simulink model "CLSfixedExample3"  (R2025b)
settings: Solver=FixedStepAuto  StartTime=0.0  StopTime=10  FixedStep=0.0005  RelTol=1e-3
undefined symbols (not defined in the file or in its folder): AVI, cfg_length, LRI, pNode_length, pPath_length, PVARP, stepsize, URI, VRP
libraries: Libs x12, Libs_unified x3
settings Model: SimulationMode=accelerator  Creator=ball907  LastModifiedBy=rfen801
settings SolverCC: AutoInsertRateTranBlk=on
settings OptimizationCC: DefaultParameterBehavior=Inlined
settings ModelReferenceCC: EnableRefExpFcnMdlSchedulingChecks=on
settings RTWCC: Toolchain=Simulink Real-Time Toolchain  BuildConfiguration=Faster Runs  CodeExecutionProfiling=on

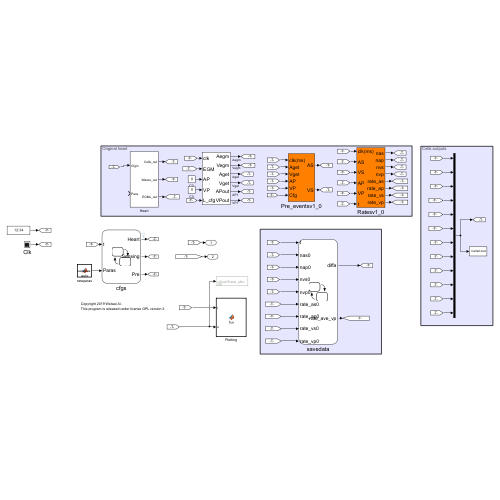
[thumbnail: Simulink's stored preview of the top-level diagram]
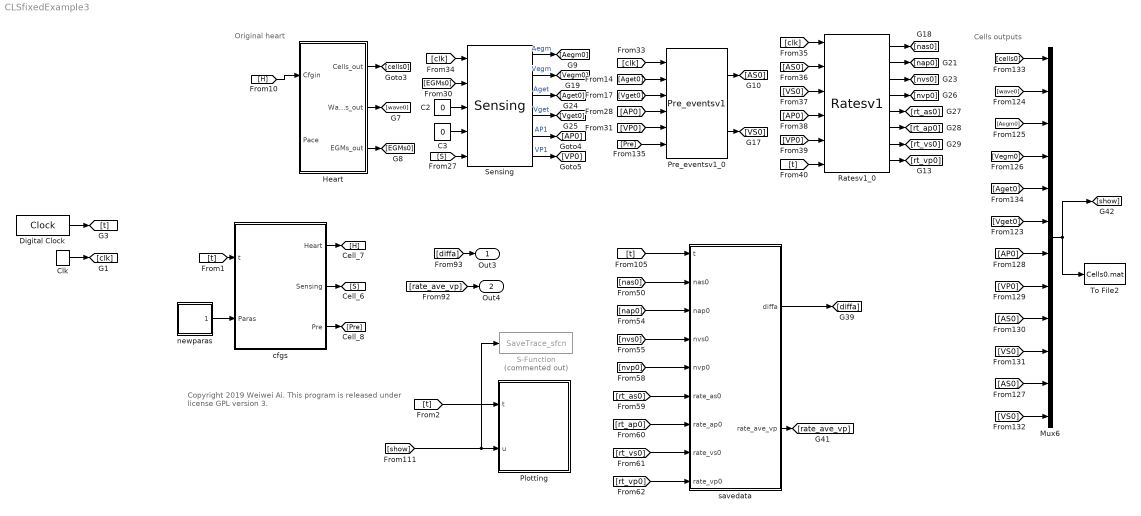
== system CLSfixedExample3 ==
  note: Cells outputs
  note: Copyright 2019 Weiwei Ai.
      | This program is released under license GPL version 3.
  note: Original heart
  C2 : Constant  Value=0
  C3 : Constant  Value=0
  Clk : DiscretePulseGenerator  PulseType=Time based  Period=1  PulseWidth=50
  Digital Clock : DigitalClock  SampleTime=stepsize
  Heart : Subsystem
  Mux6 : Mux  Inputs=12
  Plotting : MATLAB Function  TreatAsAtomicUnit=on  SystemSampleTime=stepsize*5
  Pre_eventsv1_0 : Libs_unified/Pre_eventsv1  SystemSampleTime=-1  VariantActivationTime=update diagram  EmptyChoice=off  PassThrough=off  PassThroughVariantControl=(default)  EmptyChoiceVariantControl=(default)  AllowFlexibleInterface=on  Latency=0  AutoFrameSizeCalculation=off
  Ratesv1_0 : Libs_unified/Ratesv1  SystemSampleTime=-1  VariantActivationTime=update diagram  EmptyChoice=off  PassThrough=off  PassThroughVariantControl=(default)  EmptyChoiceVariantControl=(default)  AllowFlexibleInterface=on  Latency=0  AutoFrameSizeCalculation=off
  S-Function : S-Function  Commented=on  FunctionName=SaveTrace_sfcn  Parameters=1  SFunctionDeploymentMode=off  EnableBusSupport=off
  Sensing : Libs_unified/Sensing  SystemSampleTime=-1  VariantActivationTime=update diagram  EmptyChoice=off  PassThrough=off  PassThroughVariantControl=(default)  EmptyChoiceVariantControl=(default)  AllowFlexibleInterface=on  Latency=0  AutoFrameSizeCalculation=off
  To File2 : ToFile  Filename=Cells0.mat  MatrixName=cells
      settings: Decimation=2
  cfgs : Stateflow chart  TreatAsAtomicUnit=on
  newparas : MATLAB Function  TreatAsAtomicUnit=on
  savedata : Stateflow chart  TreatAsAtomicUnit=on
  Out3 : Outport
  Out4 : Outport  Port=2
  wires:
  Sensing/6 -> [VP0]  "VP1"
  [VS0] -> Mux6/10
  [VS0] -> Ratesv1_0/3
  Pre_eventsv1_0/1 -> [AS0]
  [nap0] -> savedata/3(nap0)
  [VP0] -> Pre_eventsv1_0/5
  [AS0] -> Mux6/11
  Sensing/3 -> [Aget0]  "Aget"
  [rt_ap0] -> savedata/7(rate_ap0)
  C3/1 -> Sensing/4
  [AS0] -> Mux6/9
  Sensing/1 -> [Aegm0]  "Aegm"
  Ratesv1_0/4 -> [nvp0]
  [t] -> savedata/1(t)
  savedata/1(diffa) -> [diffa]
  Heart/3(EGMs_out) -> [EGMs0]
  [cells0] -> Mux6/1
  Pre_eventsv1_0/2 -> [VS0]
  Sensing/4 -> [Vget0]  "Vget"
  Ratesv1_0/5 -> [rt_as0]
  Ratesv1_0/3 -> [nvs0]
  [rt_vp0] -> savedata/9(rate_vp0)
  [rt_vs0] -> savedata/8(rate_vs0)
  [Aget0] -> Pre_eventsv1_0/2
  Sensing/5 -> [AP0]  "AP1"
  Ratesv1_0/1 -> [nas0]
  [diffa] -> Out3/1
  Heart/1(Cells_out) -> [cells0]
  Ratesv1_0/2 -> [nap0]
  [VP0] -> Mux6/8
  Mux6/1 -> [show], To File2/1
  [AS0] -> Ratesv1_0/2
  [AP0] -> Mux6/7
  [t] -> Ratesv1_0/6
  [Aegm0] -> Mux6/3
  [nvs0] -> savedata/4(nvs0)
  [Vget0] -> Mux6/6
  [rt_as0] -> savedata/6(rate_as0)
  [VS0] -> Mux6/12
  [AP0] -> Ratesv1_0/4
  Heart/2(Waves_out) -> [wave0]
  [clk] -> Ratesv1_0/1
  [clk] -> Pre_eventsv1_0/1
  [Pre] -> Pre_eventsv1_0/6
  [Vget0] -> Pre_eventsv1_0/3
  [wave0] -> Mux6/2
  [VP0] -> Ratesv1_0/5
  [AP0] -> Pre_eventsv1_0/4
  savedata/2(rate_ave_vp) -> [rate_ave_vp]
  C2/1 -> Sensing/3
  [S] -> Sensing/5
  [rate_ave_vp] -> Out4/1
  Ratesv1_0/7 -> [rt_vs0]
  [Vegm0] -> Mux6/4
  [clk] -> Sensing/1
  Ratesv1_0/8 -> [rt_vp0]
  [Aget0] -> Mux6/5
  [H] -> Heart/1(Cfgin)
  [nas0] -> savedata/2(nas0)
  [EGMs0] -> Sensing/2
  Sensing/2 -> [Vegm0]  "Vegm"
  Ratesv1_0/6 -> [rt_ap0]
  [nvp0] -> savedata/5(nvp0)
  cfgs/2(Sensing) -> [S]
  cfgs/3(Pre) -> [Pre]
  newparas/1(newparas) -> cfgs/2(Paras)
  cfgs/1(Heart) -> [H]
  [t] -> cfgs/1(t)
  Digital Clock/1 -> [t]
  Clk/1 -> [clk]
  [show] -> S-Function/1, Plotting/2(u)
  [t] -> Plotting/1(t)

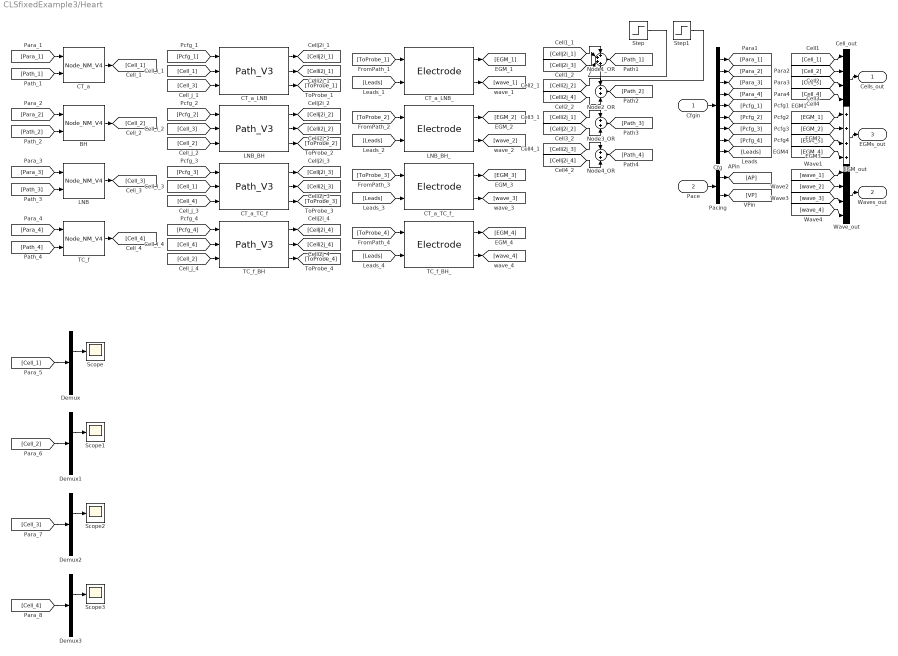
== system CLSfixedExample3/Heart ==
  Cfgin : Inport
  Pace : Inport  Port=2
  BH : Libs/Node_NM_V4  SystemSampleTime=-1  VariantActivationTime=update diagram  EmptyChoice=off  PassThrough=off  PassThroughVariantControl=(default)  EmptyChoiceVariantControl=(default)  AllowFlexibleInterface=on  Latency=0  AutoFrameSizeCalculation=off
  CT_a : Libs/Node_NM_V4  SystemSampleTime=-1  VariantActivationTime=update diagram  EmptyChoice=off  PassThrough=off  PassThroughVariantControl=(default)  EmptyChoiceVariantControl=(default)  AllowFlexibleInterface=on  Latency=0  AutoFrameSizeCalculation=off
  CT_a_LNB : Libs/Path_V3  SystemSampleTime=-1  VariantActivationTime=update diagram  EmptyChoice=off  PassThrough=off  PassThroughVariantControl=(default)  EmptyChoiceVariantControl=(default)  AllowFlexibleInterface=on  Latency=0  AutoFrameSizeCalculation=off
  CT_a_LNB_ : Libs/Electrode  SystemSampleTime=-1  VariantActivationTime=update diagram  EmptyChoice=off  PassThrough=off  PassThroughVariantControl=(default)  EmptyChoiceVariantControl=(default)  AllowFlexibleInterface=on  Latency=0  AutoFrameSizeCalculation=off
  CT_a_TC_f : Libs/Path_V3  SystemSampleTime=-1  VariantActivationTime=update diagram  EmptyChoice=off  PassThrough=off  PassThroughVariantControl=(default)  EmptyChoiceVariantControl=(default)  AllowFlexibleInterface=on  Latency=0  AutoFrameSizeCalculation=off
  CT_a_TC_f_ : Libs/Electrode  SystemSampleTime=-1  VariantActivationTime=update diagram  EmptyChoice=off  PassThrough=off  PassThroughVariantControl=(default)  EmptyChoiceVariantControl=(default)  AllowFlexibleInterface=on  Latency=0  AutoFrameSizeCalculation=off
  Cell_out : Mux
  Cfg : Demux  Outputs=[50,50,50,50,11,11,11,11,28]
  Demux{,1..3} (4 alike) : Demux  Outputs=5
  EGM_out : Sum  Inputs=4
  LNB : Libs/Node_NM_V4  SystemSampleTime=-1  VariantActivationTime=update diagram  EmptyChoice=off  PassThrough=off  PassThroughVariantControl=(default)  EmptyChoiceVariantControl=(default)  AllowFlexibleInterface=on  Latency=0  AutoFrameSizeCalculation=off
  LNB_BH : Libs/Path_V3  SystemSampleTime=-1  VariantActivationTime=update diagram  EmptyChoice=off  PassThrough=off  PassThroughVariantControl=(default)  EmptyChoiceVariantControl=(default)  AllowFlexibleInterface=on  Latency=0  AutoFrameSizeCalculation=off
  LNB_BH_ : Libs/Electrode  SystemSampleTime=-1  VariantActivationTime=update diagram  EmptyChoice=off  PassThrough=off  PassThroughVariantControl=(default)  EmptyChoiceVariantControl=(default)  AllowFlexibleInterface=on  Latency=0  AutoFrameSizeCalculation=off
  Node1_OR : Sum  Inputs=4
  Node2_OR : Sum  Inputs=2
  Node3_OR : Sum  Inputs=2
  Node4_OR : Sum  Inputs=2
  Pacing : Demux  Outputs=2
  Scope{,1..3} (4 alike) : Scope
      Scope settings: ActiveDisplayYMinimum=-14.055953139718371  ActiveDisplayYMaximum=126.50357825746536
      Scope1 settings: ActiveDisplayYMinimum=-16.387499999999996  ActiveDisplayYMaximum=147.48749999999998
      Scope2 settings: ActiveDisplayYMinimum=-16.387499999999996  ActiveDisplayYMaximum=147.48749999999998  DataLoggingVariableName=ScopeData2
      Scope3 settings: ActiveDisplayYMinimum=-14.055953139718371  ActiveDisplayYMaximum=126.50357825746536  DataLoggingVariableName=ScopeData3
  Step : Step  Time=3.32  After=120  SampleTime=0
  Step1 : Step  Time=3.36  After=-120  SampleTime=0
  TC_f : Libs/Node_NM_V4  SystemSampleTime=-1  VariantActivationTime=update diagram  EmptyChoice=off  PassThrough=off  PassThroughVariantControl=(default)  EmptyChoiceVariantControl=(default)  AllowFlexibleInterface=on  Latency=0  AutoFrameSizeCalculation=off
  TC_f_BH : Libs/Path_V3  SystemSampleTime=-1  VariantActivationTime=update diagram  EmptyChoice=off  PassThrough=off  PassThroughVariantControl=(default)  EmptyChoiceVariantControl=(default)  AllowFlexibleInterface=on  Latency=0  AutoFrameSizeCalculation=off
  TC_f_BH_ : Libs/Electrode  SystemSampleTime=-1  VariantActivationTime=update diagram  EmptyChoice=off  PassThrough=off  PassThroughVariantControl=(default)  EmptyChoiceVariantControl=(default)  AllowFlexibleInterface=on  Latency=0  AutoFrameSizeCalculation=off
  Wave_out : Mux
  Cells_out : Outport
  Waves_out : Outport  Port=2
  EGMs_out : Outport  Port=3
  wires:
  [wave_4] -> Wave_out/4
  [wave_3] -> Wave_out/3
  [wave_2] -> Wave_out/2
  [wave_1] -> Wave_out/1
  [EGM_4] -> EGM_out/4
  [EGM_3] -> EGM_out/3
  [EGM_2] -> EGM_out/2
  [EGM_1] -> EGM_out/1
  [Cell_4] -> Cell_out/4
  [Cell_3] -> Cell_out/3
  [Cell_2] -> Cell_out/2
  [Cell_1] -> Cell_out/1
  Wave_out/1 -> Waves_out/1
  EGM_out/1 -> EGMs_out/1
  Cell_out/1 -> Cells_out/1
  Pacing/2 -> [VP]
  Pacing/1 -> [AP]
  Cfg/9 -> [Leads]
  Cfg/8 -> [Pcfg_4]
  Cfg/7 -> [Pcfg_3]
  Cfg/6 -> [Pcfg_2]
  Cfg/5 -> [Pcfg_1]
  Cfg/4 -> [Para_4]
  Cfg/3 -> [Para_3]
  Cfg/2 -> [Para_2]
  Cfg/1 -> [Para_1]
  Pace/1 -> Pacing/1
  Cfgin/1 -> Cfg/1
  Node4_OR/1 -> [Path_4]
  [Cellj2i_4] -> Node4_OR/2
  [Celli2j_3] -> Node4_OR/1
  Node3_OR/1 -> [Path_3]
  [Cellj2i_2] -> Node3_OR/2
  [Celli2j_1] -> Node3_OR/1
  Node2_OR/1 -> [Path_2]
  [Celli2j_4] -> Node2_OR/2
  [Celli2j_2] -> Node2_OR/1
  Node1_OR/1 -> [Path_1]
  [Cellj2i_3] -> Node1_OR/2
  [Cellj2i_1] -> Node1_OR/1
  [Leads] -> TC_f_BH_/2
  [ToProbe_4] -> TC_f_BH_/1
  TC_f_BH_/2 -> [wave_4]
  TC_f_BH_/1 -> [EGM_4]
  [Leads] -> CT_a_TC_f_/2
  [ToProbe_3] -> CT_a_TC_f_/1
  CT_a_TC_f_/2 -> [wave_3]
  CT_a_TC_f_/1 -> [EGM_3]
  [Leads] -> LNB_BH_/2
  [ToProbe_2] -> LNB_BH_/1
  LNB_BH_/2 -> [wave_2]
  LNB_BH_/1 -> [EGM_2]
  [Leads] -> CT_a_LNB_/2
  [ToProbe_1] -> CT_a_LNB_/1
  CT_a_LNB_/2 -> [wave_1]
  CT_a_LNB_/1 -> [EGM_1]
  [Cell_2] -> TC_f_BH/3
  [Cell_4] -> TC_f_BH/2
  [Pcfg_4] -> TC_f_BH/1
  TC_f_BH/3 -> [ToProbe_4]
  TC_f_BH/2 -> [Celli2j_4]
  TC_f_BH/1 -> [Cellj2i_4]
  [Cell_4] -> CT_a_TC_f/3
  [Cell_1] -> CT_a_TC_f/2
  [Pcfg_3] -> CT_a_TC_f/1
  CT_a_TC_f/3 -> [ToProbe_3]
  CT_a_TC_f/2 -> [Celli2j_3]
  CT_a_TC_f/1 -> [Cellj2i_3]
  [Cell_2] -> LNB_BH/3
  [Cell_3] -> LNB_BH/2
  [Pcfg_2] -> LNB_BH/1
  LNB_BH/3 -> [ToProbe_2]
  LNB_BH/2 -> [Celli2j_2]
  LNB_BH/1 -> [Cellj2i_2]
  [Cell_3] -> CT_a_LNB/3
  [Cell_1] -> CT_a_LNB/2
  [Pcfg_1] -> CT_a_LNB/1
  CT_a_LNB/3 -> [ToProbe_1]
  CT_a_LNB/2 -> [Celli2j_1]
  CT_a_LNB/1 -> [Cellj2i_1]
  [Path_4] -> TC_f/2
  [Para_4] -> TC_f/1
  TC_f/1 -> [Cell_4]
  [Path_3] -> LNB/2
  [Para_3] -> LNB/1
  LNB/1 -> [Cell_3]
  [Path_2] -> BH/2
  [Para_2] -> BH/1
  BH/1 -> [Cell_2]
  [Path_1] -> CT_a/2
  [Para_1] -> CT_a/1
  CT_a/1 -> [Cell_1]
  [Cell_1] -> Demux/1
  Demux/2 -> Scope/1
  Demux1/2 -> Scope1/1
  [Cell_2] -> Demux1/1
  [Cell_3] -> Demux2/1
  Demux2/2 -> Scope2/1
  Demux3/2 -> Scope3/1
  [Cell_4] -> Demux3/1
  Step/1 -> Node1_OR/3
  Step1/1 -> Node1_OR/4

== stateflow chart CLSfixedExample3/cfgs ==
  settings: executeAtInitialization=1
  state Ini
  state wait
  Ini -> wait : [t>800]{pUpdate(Paras);}
  (default) -> Ini : {Sensing=Scfgf;[Pre]=Precfg;...
      |  [Heart] =LoadInit;}
  data: Scfg function_output; Preout function_output; LRI parameter; AVI parameter; VRP parameter; URI parameter; PVARP parameter; Parasin function_input; pNode_length parameter; pPath_length parameter; Hcfg function_output; cfg_length parameter; Heart output; Sensing output; t input; Paras input; Pre output
  function Scfg= Scfgf:
    | function Scfg= Scfgf
    | 
    | %% desired
    | xa=1;
    | xc=0.05;
    | xc1=0.1;
    | xd=1;
    | xe=0.1;
    | avd=100;
    | vad=100;
    | uni_a=1;
    | Sens_a=0.6;
    | Amp_ap=500;
    | uni_v=1;
    | Sens_v=2.8;
    | Amp_vp=500;
    | 
    | Scfg=[xa xc xc1 xd xe avd vad uni_a Sens_a Amp_ap uni_v Sens_v Amp_vp]';
    | 
    | end
  function Preout = Precfg:
    | function Preout = Precfg
    | % 
    | % LRI=1000;
    | % AVI=170;
    | % URI=500;
    | % VRP=230;
    | % PVARP=250;
    | Preout=[VRP PVARP];
    | 
    | end
  function pUpdate(Parasin):
    | %% Get the index of the parameter
    | function pUpdate(Parasin)
    | %#codegen
    | coder.extrinsic('evalin');
    | coder.extrinsic('assignin');
    | Nodein=zeros(1,pNode_length); % The total number of cell cfg ports
    | Nodein=evalin('base', 'pNode');
    | Pathin=zeros(1,pPath_length); % The total number of path cfg ports
    | Pathin=evalin('base', 'pPath');
    | for n=1:pNode_length
    |     m=Nodein(n);
    |     Heart(m)=Parasin(n);
    | end
    | 
    | for n=1:pPath_length
    |     m=Pathin(n);
    |     nn=n+length(Nodein);
    |     Heart(m)=Parasin(nn);
    | end
    | 
    | assignin('base', 'Params', Parasin);
    | 
    | end
  function Hcfg   = LoadInit:
    | function Hcfg   = LoadInit
    | %#codegen
    | coder.extrinsic('evalin');
    | Hcfg1=zeros(1,cfg_length); % The total number of cfg ports
    | Hcfg1=evalin('base', 'cfgdata');
    | Hcfg=Hcfg1';
    | end

== matlab function CLSfixedExample3/Plotting ==
  data: t input; u input
function fcn(t,u)
%coder.extrinsic('evalin')
coder.extrinsic('updateGUIplots')
fun = 'updateGUIplots';
updateGUIplots(t,u)
%feval(fun,t,u)
end

== matlab function CLSfixedExample3/newparas ==
  data: newparas output; paras_length parameter

function newparas= auto(paras_length)

coder.extrinsic('evalin');
%par_length = evalin('base','paras_length')
newparas=zeros(1,paras_length); % The total number of cell cfg ports
newparas=evalin('base', 'pp');

end

== stateflow chart CLSfixedExample3/savedata ==
  settings: executeAtInitialization=1
  state termi
  state difa
  state Ini
  difa -> termi [order 1] : [rate_ave_a0>=60]/{coder.extrinsic('assignin');diffa=rate_ave_a1-rate_ave_a0;assignin('base', 'diffa', diffa);}
  (default) -> Ini : {rate_ave_vp=0; diffa=0;}
  Ini -> difa : [t>=29998]{coder.extrinsic('assignin','mean');...
      | assignin('base', 'nas0', nas0);assignin('base', 'nap0', nap0);assignin('base', 'nvs0', nvs0);assignin('base', 'nvp0', nvp0);...
      | assignin('base', 'rate_as0', rate_as0);assignin('base', 'rate_ap0', rate_ap0);assignin('base', 'rate_vs0', rate_vs0);assignin('base', 'rate_vp0', rate_vp0);...
      | rate_ave_vp=mean(rate_vp0(2,1:nvp0));assignin('base', 'rate_ave_vp', rate_ave_vp);...
      | rate_ave_a1=0;rate_ave_a0=0;rate_ave_a0=mean(rate_as0(2,1:nas0));rate_ave_a1=zeros(size(rate_ave_a0),like=rate_ave_a0);}
  difa -> termi [order 2] : [rate_ave_a0<60]/{coder.extrinsic('assignin');diffa=rate_ave_a1-60;assignin('base', 'diffa', diffa);}
  data: t input; nas0 input; nap0 input; nvs0 input; nvp0 input; rate_as0 input; rate_ap0 input; rate_vs0 input; rate_vp0 input; diffa output double; rate_ave_vp output double; rate_ave_a0 local double; rate_ave_a1 local double
